simulink model "PTODi_SpdCoord"  (R2016b)
settings: configuration reference "CodeGenConfigSet" (kept outside this file)
settings Model: Creator=lenovo  LastModifiedBy=lenovo
settings ConfigSetRef: SourceLocation=Base Workspace

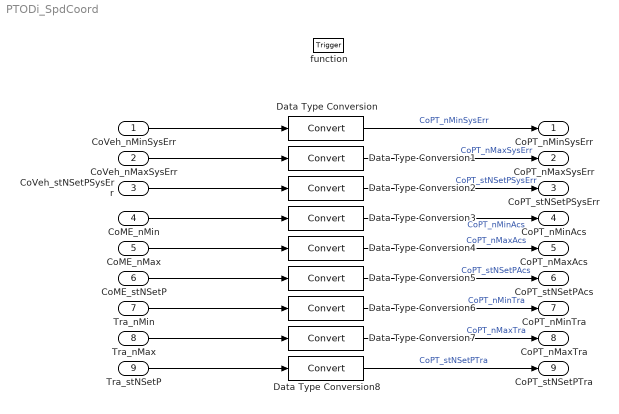
== system PTODi_SpdCoord ==
  CoVeh_nMinSysErr : Inport  Tag=rpm  Description=Minimum speed limitation in case of system errors  OutMin=-12000  OutMax=12000  OutDataTypeStr=EngSpeed_rpm
  CoVeh_nMaxSysErr : Inport  Tag=rpm  Description=Maximum speed limitation in case of system errors  Port=2  OutMin=-12000  OutMax=12000  OutDataTypeStr=EngSpeed_rpm
  CoVeh_stNSetPSysErr : Inport  Description=Status word which defines the conversion of the system error speed requirements  Port=3  OutMin=0  OutMax=255  OutDataTypeStr=State_uint8
  CoME_nMin : Inport  Tag=rpm  Description=Minimum low-idle speed requirement of accessories  Port=4  OutMin=-12000  OutMax=12000  OutDataTypeStr=EngSpeed_rpm
  CoME_nMax : Inport  Tag=rpm  Description=Maximum engine speed limit of accessories  Port=5  OutMin=-12000  OutMax=12000  OutDataTypeStr=EngSpeed_rpm
  CoME_stNSetP : Inport  Description=Status: Nature of low-idle speed increase  Port=6  OutMin=0  OutMax=255  OutDataTypeStr=State_uint8
  Tra_nMin : Inport  Tag=rpm  Description=Minimum engine speed for gearbox  Port=7  OutMin=-6000  OutMax=6000  OutDataTypeStr=EngSpeed_rpm
  Tra_nMax : Inport  Tag=rpm  Description=Maximum engine speed for gearbox  Port=8  OutMin=-6000  OutMax=11000  OutDataTypeStr=EngSpeed_rpm
  Tra_stNSetP : Inport  Description=Status for current set point engine speed requirement  Port=9  OutMin=0  OutMax=255  OutDataTypeStr=State_uint8
  function : TriggerPort  TriggerType=function-call  VariantControl=Variant
  Data Type Conversion{,1..8} (9 alike) : DataTypeConversion
  CoPT_nMinSysErr : Outport  Tag=rpm  Description=Application parameter for Minimum engine speed demand while system error  OutMin=0  OutMax=6000  OutDataTypeStr=EngSpeed_rpm
  CoPT_nMaxSysErr : Outport  Tag=rpm  Description=Application parameter for maximum engine speed demand while system error  Port=2  OutMin=0  OutMax=6000  OutDataTypeStr=EngSpeed_rpm
  CoPT_stNSetPSysErr : Outport  Description=Application parameter for state of low idle speed request while system error  Port=3  OutMin=0  OutMax=255  OutDataTypeStr=State_uint8
  CoPT_nMinAcs : Outport  Tag=rpm  Description=Application parameter for Minimum engine speed demand of Accessories  Port=4  OutMin=0  OutMax=6000  OutDataTypeStr=EngSpeed_rpm
  CoPT_nMaxAcs : Outport  Tag=rpm  Description=Application parameter for maximum engine speed  Port=5  OutMin=0  OutMax=6000  OutDataTypeStr=EngSpeed_rpm
  CoPT_stNSetPAcs : Outport  Description=Application parameter for state of low idle speed request of accessories  Port=6  OutMin=0  OutMax=255  OutDataTypeStr=State_uint8
  CoPT_nMinTra : Outport  Tag=rpm  Description=Application parameter for Minimum engine speed demand of transmission  Port=7  OutMin=0  OutMax=6000  OutDataTypeStr=EngSpeed_rpm
  CoPT_nMaxTra : Outport  Tag=rpm  Description=Application parameter for maximum engine speed demand of transmission  Port=8  OutMin=0  OutMax=6000  OutDataTypeStr=EngSpeed_rpm
  CoPT_stNSetPTra : Outport  Description=Application parameter for state of low idle speed request of transmission  Port=9  OutMin=0  OutMax=255  OutDataTypeStr=State_uint8
  wires:
  Data Type Conversion/1 -> CoPT_nMinSysErr/1  "CoPT_nMinSysErr"
  Data Type Conversion1/1 -> CoPT_nMaxSysErr/1  "CoPT_nMaxSysErr"
  Data Type Conversion2/1 -> CoPT_stNSetPSysErr/1  "CoPT_stNSetPSysErr"
  Data Type Conversion3/1 -> CoPT_nMinAcs/1  "CoPT_nMinAcs"
  Data Type Conversion4/1 -> CoPT_nMaxAcs/1  "CoPT_nMaxAcs"
  Data Type Conversion5/1 -> CoPT_stNSetPAcs/1  "CoPT_stNSetPAcs"
  Data Type Conversion6/1 -> CoPT_nMinTra/1  "CoPT_nMinTra"
  Data Type Conversion7/1 -> CoPT_nMaxTra/1  "CoPT_nMaxTra"
  Data Type Conversion8/1 -> CoPT_stNSetPTra/1  "CoPT_stNSetPTra"
  CoVeh_nMinSysErr/1 -> Data Type Conversion/1
  CoVeh_nMaxSysErr/1 -> Data Type Conversion1/1
  CoVeh_stNSetPSysErr/1 -> Data Type Conversion2/1
  CoME_nMin/1 -> Data Type Conversion3/1
  CoME_nMax/1 -> Data Type Conversion4/1
  CoME_stNSetP/1 -> Data Type Conversion5/1
  Tra_nMin/1 -> Data Type Conversion6/1
  Tra_nMax/1 -> Data Type Conversion7/1
  Tra_stNSetP/1 -> Data Type Conversion8/1
